simulink model "hybrid_fuzzy"  (R2020a)
settings: Solver=VariableStepAuto  StartTime=0.0  StopTime=1  RelTol=1e-3
undefined symbols (not defined in the file): DiscIntNeverNeededParam, LowerLimit, UpperLimit
libraries: powerlib x44, powerlib_extras x7, powerlib_meascontrol x6, fuzblock x2, re_lib x2, simulink x1, sdolib x1
settings Model: SimulationMode=accelerator  Creator=vardh  LastModifiedBy=vardh

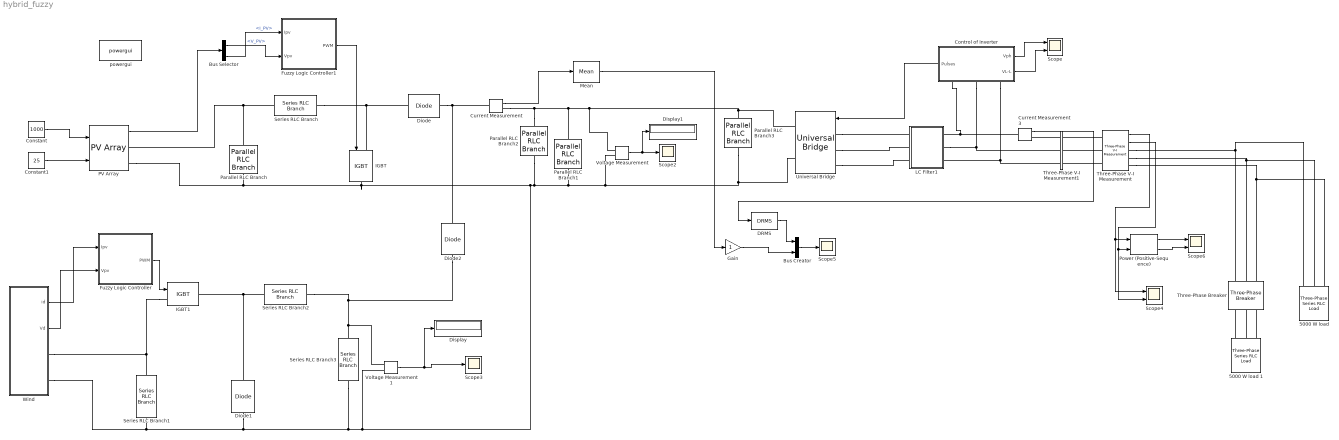
== system hybrid_fuzzy ==
  "5000 W load " : powerlib/Elements/Three-Phase Series RLC Load  LConnTagsString=A|B|C  Configuration=Y (grounded)  NominalVoltage=440  Vabc=[1e3 1e3 1e3]  Vabcp=[1e3 1e3 1e3]  NominalFrequency=50  UnbalancedPower=off  ActivePower=300e3  InductivePower=0  CapacitivePower=0  Pabc=[10e3 9e3 11e3]  QLabc=[100 90 110]  QCabc=[100 90 110]  Pabcp=[10e3 9e3 11e3]  QLabcp=[100 90 110]  QCabcp=[100 90 110]  Measurements=Branch voltages and currents  LoadType=constant PQ
  5000 W load 1 : powerlib/Elements/Three-Phase Series RLC Load  LConnTagsString=A|B|C  Configuration=Y (grounded)  NominalVoltage=440  Vabc=[1e3 1e3 1e3]  Vabcp=[1e3 1e3 1e3]  NominalFrequency=50  UnbalancedPower=off  ActivePower=300e3  InductivePower=0  CapacitivePower=0  Pabc=[10e3 9e3 11e3]  QLabc=[100 90 110]  QCabc=[100 90 110]  Pabcp=[10e3 9e3 11e3]  QLabcp=[100 90 110]  QCabcp=[100 90 110]  Measurements=Branch voltages and currents  LoadType=constant PQ
  Bus Creator : BusCreator  Inputs=2
  Bus Selector : BusSelector  OutputSignals=V_PV,I_PV
  Constant : Constant  Value=1000
  Constant1 : Constant  Value=25
  Control of Inverter : Subsystem
      settings: PortSchema="{\"entries\":[{\"content\":{\"sides\":[{\"content\":{\"connectorIds\":[\"Out2\",\"Out3\"]},\"type\":\"ConnectorPlacement.EquallySpacedRectSide\",\"uuid\":\"6e599ea3-178d-4f76-bb70-cdc4ed3450cd\"},{\"content\":{\"connectorIds\":[\"Out1\"],\"side\":\"RIGHT\"},\"type\":\"ConnectorPlacement.EquallySpacedRectSide\",\"uuid\":\"1f076554-0d11-4549-8e28-a9b47f6feaf3\"},{\"content\":{\"connectorIds\":[],\"side\":\"TOP\"},\"type\":\"ConnectorPlacement.EquallySpacedRectSide\",\"uuid\":\"86982356-7389-48f3-89f0-a125c4c11ea8\"},{\"content\":{\"connectorIds\":[\"RConn1\",\"RConn2\",\"RConn3\"],\"side\":\"BOTTOM\"},\"type\":\"ConnectorPlacement.EquallySpacedRectSide\",\"uuid\":\"f2c41feb-d46e-404e-b0df-a8035424fc9b\"}]},\"type\":\"ConnectorPlacement.EquallySpacedConnector\",\"uuid\":\"7cdef0cd-0041-4714-b9be-c27206ef597d\"}],\"packageUris\":[\"http://schema.mathworks.com/mf0/Connector/19700101\"],\"version\":\"1.0\"}"
  Current Measurement : powerlib/Measurements/Current Measurement  PhasorSimulation=off  OutputType=Complex  PSBequivalent=0
  Current Measurement3 : powerlib/Measurements/Current Measurement  PhasorSimulation=off  OutputType=Complex  PSBequivalent=0
  DRMS : sdolib/RMS Blocks/DRMS  Ts=5e-6
      settings: SourceProductBaseCode=SO
  Diode : powerlib/Power Electronics/Diode  Ron=0.001  Lon=0  Vf=0.8  IC=0  UseSnubber=0  Rs=500  Cs=250e-9  Measurements=off
  Diode1 : powerlib/Power Electronics/Diode  Ron=0.001  Lon=0  Vf=0.8  IC=0  UseSnubber=0  Rs=500  Cs=250e-9  Measurements=off
  Diode2 : powerlib/Power Electronics/Diode  Ron=0.001  Lon=0  Vf=0.8  IC=0  UseSnubber=0  Rs=500  Cs=250e-9  Measurements=off
  Display : Display
  Display1 : Display
  Fuzzy Logic Controller : Subsystem
  Fuzzy Logic Controller1 : Subsystem
  Gain : Gain
  IGBT : powerlib/Power Electronics/IGBT  Ron=0.001  Lon=0  Vf=1  Tf=1e-6  Tt=2e-6  IC=0  Rs=1e5  Cs=inf  Measurements=off
  IGBT1 : powerlib/Power Electronics/IGBT  Ron=0.001  Lon=0  Vf=1  Tf=1e-6  Tt=2e-6  IC=0  Rs=1e5  Cs=inf  Measurements=off
  LC Filter1 : Subsystem
  Mean : powerlib_meascontrol/Measurements/Mean  Freq=60  Vinit=0  Ts=5e-6
  PV Array : re_lib/Solar/PV Array  Npar=1  Nser=9  PlotType=one module @ 25 deg.C & specified irradiances  S_vec="[ 1000  800  600 ]"  Temp_C_vec="[ 45 25  ]"  ModuleName=Kyocera Solar KC200GT  PlotWhenSelected=off  Pm=200.143  Ncell=54  Voc=32.9  Isc=8.21  Vm=26.3  Im=7.61  beta_Voc_pc=-0.35502  alpha_Isc_pc=0.06  beta_Voc=-0.1168  alpha_Isc=0.004926  IL=8.2288  I0=2.3246e-10  nI=0.97736  Rsh=150.6921  Rs=0.34483  RobustModel=off  RobustCellTemperature=25  BAL=on  Tc=1e-6  Tfilter=5e-5
  Parallel RLC Branch : powerlib/Elements/Parallel RLC Branch  LConnTagsString=a  RConnTagsString=__new0  BranchType=C  Resistance=1  Inductance=1e-3  SetiL0=off  InitialCurrent=0  Capacitance=10e-6  Setx0=off  InitialVoltage=0  Measurements=None
  Parallel RLC Branch1 : powerlib/Elements/Parallel RLC Branch  LConnTagsString=a  RConnTagsString=__new0  BranchType=C  Resistance=1  Inductance=1e-3  SetiL0=off  InitialCurrent=0  Capacitance=10000e-6  Setx0=off  InitialVoltage=0  Measurements=None
  Parallel RLC Branch2 : powerlib/Elements/Parallel RLC Branch  LConnTagsString=a  RConnTagsString=__new0  BranchType=R  Resistance=30  Inductance=1e-3  SetiL0=off  InitialCurrent=0  Capacitance=1e-6  Setx0=off  InitialVoltage=0  Measurements=None
  Parallel RLC Branch3 : powerlib/Elements/Parallel RLC Branch  LConnTagsString=a  RConnTagsString=__new0  BranchType=R  Resistance=30  Inductance=1e-3  SetiL0=off  InitialCurrent=0  Capacitance=1e-6  Setx0=off  InitialVoltage=0  Measurements=None
  Power (Positive-Sequence) : powerlib_meascontrol/Measurements/Power (Positive-Sequence)  Freq=60  Vinit=[0, 0]  Iinit=[0, 0]  Ts=5e-6
      settings: SourceProductBaseCode=PS
  Scope : Scope  NumInputPorts=2
  Scope2 : Scope
  Scope3 : Scope
  Scope4 : Scope  NumInputPorts=2
  Scope5 : Scope
  Scope6 : Scope  NumInputPorts=2
  Series RLC Branch : powerlib/Elements/Series RLC Branch  LConnTagsString=__new0  RConnTagsString=__new0  BranchType=L  Resistance=1  Inductance=100e-3  SetiL0=off  InitialCurrent=0  Capacitance=1e-6  Setx0=off  InitialVoltage=0  Measurements=None
  Series RLC Branch1 : powerlib/Elements/Series RLC Branch  LConnTagsString=__new0  RConnTagsString=__new0  BranchType=C  Resistance=1  Inductance=1e-3  SetiL0=off  InitialCurrent=0  Capacitance=10e-6  Setx0=off  InitialVoltage=0  Measurements=None
  Series RLC Branch2 : powerlib/Elements/Series RLC Branch  LConnTagsString=__new0  RConnTagsString=__new0  BranchType=L  Resistance=1  Inductance=100e-3  SetiL0=off  InitialCurrent=0  Capacitance=1e-6  Setx0=off  InitialVoltage=0  Measurements=None
  Series RLC Branch3 : powerlib/Elements/Series RLC Branch  LConnTagsString=__new0  RConnTagsString=__new0  BranchType=R  Resistance=50  Inductance=1e-3  SetiL0=off  InitialCurrent=0  Capacitance=1e-6  Setx0=off  InitialVoltage=0  Measurements=None
  Three-Phase V-I Measurement : powerlib/Measurements/Three-Phase V-I Measurement  VoltageMeasurement=phase-to-phase  SetLabelV=off  LabelV=Vabc  Vpu=off  VpuLL=off  CurrentMeasurement=yes  SetLabelI=off  LabelI=Iabc  Ipu=off  Pbase=100e6  Vbase=500e3  OutputType=Complex  PhasorSimulation=off  PSBequivalent=0
  Three-Phase V-I Measurement1 : powerlib/Measurements/Three-Phase V-I Measurement  VoltageMeasurement=no  SetLabelV=off  LabelV=Vabc  Vpu=off  VpuLL=off  CurrentMeasurement=no  SetLabelI=off  LabelI=Iabc  Ipu=off  Pbase=100e6  Vbase=500e3  OutputType=Complex  PhasorSimulation=off  PSBequivalent=0
  Three-Phase Breaker : powerlib/Elements/Three-Phase Breaker  InitialState=open  SwitchA=on  SwitchB=on  SwitchC=on  SwitchTimes="[1/60  5/60]"  External=off  BreakerResistance=0.01  SnubberResistance=1e6  SnubberCapacitance=inf  Measurements=None
  Universal Bridge : powerlib/Power Electronics/Universal Bridge  Arms=3  SnubberResistance=1e5  SnubberCapacitance=inf  Device=IGBT / Diodes  Ron=1e-3  Lon=0  ForwardVoltages="[  0  0  ]"  ForwardVoltage=0  GTOparameters=[ 10e-6 , 20e-6 ]  IGBTparameters=[ 1e-6 , 2e-6 ]  Measurements=None  Measurements_2=None  converterType=Rectifier
  Voltage Measurement : powerlib/Measurements/Voltage Measurement  PhasorSimulation=off  OutputType=Complex  PSBequivalent=0
  Voltage Measurement1 : powerlib/Measurements/Voltage Measurement  PhasorSimulation=off  OutputType=Complex  PSBequivalent=0
  Wind : Subsystem
  powergui : powerlib/powergui  Priority=1  SimulationMode=Discrete  SampleTime=5e-6  frequency=60  Iterations=50  frequencyindice=0  Pbase=100e6  ErrMax=1e-4  UnitsV=kV  UnitsW=MW  buscounter=0  FunctionMessages=off  echomessages=off  EnableUseOfTLC=off  CurrentSourceSwitches=off  DisableSnubberDevices=off  DisableRonSwitches=off  DisableVfSwitches=off  DisplayEquations=off  AutomaticDiscreteSolvers=off  SolverType=Tustin/Backward Euler (TBE)  Interpol=off  ExternalGateDelay=off  methode=off  Ts=100  x0status=blocks  SPID=on  SwTol=0  HookPort=off  NonlinearTolerance=1e-4  nMaxIteration=100  ContinueOnMaxIteration=off  RestoreLinks=warning  ResistiveCurrentMeasurement=off  Frange=[0:2:500]  Ylog=off  Xlog=on  ShowGrid=off  save=off  variable=ZData  structure=0  ZoomFFT=off  StartTime=0.0  cycles=1  DisplayStyle=1  fundamental=60  FreqAxis=off  MaxFrequency=1000  frequencyindicesteady=1  RmsSteady=1  display=off
  wires:
  Bus Selector/2 -> Fuzzy Logic Controller1/1(Ipv)  "<I_PV>"
  Wind/2(Vd) -> Fuzzy Logic Controller/2(Vpv)
  Fuzzy Logic Controller1/1(PWM) -> IGBT/1
  Wind/1(id) -> Fuzzy Logic Controller/1(Ipv)
  Power (Positive-Sequence)/1 -> Scope6/1
  Bus Selector/1 -> Fuzzy Logic Controller1/2(Vpv)  "<V_PV>"
  Voltage Measurement/1 -> Display1/1, Scope2/1
  Current Measurement/1 -> Mean/1
  Control of Inverter/3(VL-L) -> Scope/2
  Fuzzy Logic Controller/1(PWM) -> IGBT1/1
  PV Array/1 -> Bus Selector/1
  Mean/1 -> Gain/1
  Current Measurement3/1 -> DRMS/1
  Three-Phase V-I Measurement/1 -> Scope4/1, Power (Positive-Sequence)/1
  Control of Inverter/1(Pulses) -> Universal Bridge/1
  Control of Inverter/2(Vph) -> Scope/1
  Power (Positive-Sequence)/2 -> Scope6/2
  Constant1/1 -> PV Array/2
  Constant/1 -> PV Array/1
  Bus Creator/1 -> Scope5/1
  Gain/1 -> Bus Creator/2
  Voltage Measurement1/1 -> Display/1, Scope3/1
  Three-Phase V-I Measurement/2 -> Scope4/2, Power (Positive-Sequence)/2
  DRMS/1 -> Bus Creator/1
  connections:
  LC Filter1/RConn3 -- Control of Inverter/RConn1 -- Three-Phase V-I Measurement1/RConn3
  Diode1/LConn1 -- Parallel RLC Branch/RConn1 -- PV Array/RConn2 -- IGBT/RConn1 -- Parallel RLC Branch1/RConn1 -- Parallel RLC Branch3/RConn1 -- Universal Bridge/RConn2 -- Voltage Measurement/LConn2 -- Parallel RLC Branch2/RConn1 -- Voltage Measurement1/LConn2 -- Series RLC Branch3/RConn1 -- Wind/RConn2 -- Series RLC Branch1/RConn1
  IGBT1/LConn1 -- Series RLC Branch1/LConn1 -- Wind/RConn1
  Voltage Measurement1/LConn1 -- Series RLC Branch2/RConn1 -- Diode2/LConn1 -- Series RLC Branch3/LConn1
  Series RLC Branch/LConn1 -- PV Array/RConn1 -- Parallel RLC Branch/LConn1
  Three-Phase V-I Measurement/RConn1 -- Three-Phase Breaker/RConn1 -- "5000 W load "/LConn1
  IGBT1/RConn1 -- Diode1/RConn1 -- Series RLC Branch2/LConn1
  Three-Phase Breaker/RConn2 -- "5000 W load "/LConn2 -- Three-Phase V-I Measurement/RConn2
  LC Filter1/RConn2 -- Control of Inverter/RConn2 -- Three-Phase V-I Measurement1/RConn2
  Current Measurement/LConn1 -- Diode/RConn1 -- Diode2/RConn1
  Parallel RLC Branch2/LConn1 -- Current Measurement/RConn1 -- Parallel RLC Branch3/LConn1 -- Universal Bridge/RConn1 -- Voltage Measurement/LConn1 -- Parallel RLC Branch1/LConn1
  LC Filter1/RConn1 -- Current Measurement3/LConn1 -- Control of Inverter/RConn3
  Three-Phase Breaker/RConn3 -- "5000 W load "/LConn3 -- Three-Phase V-I Measurement/RConn3
  Series RLC Branch/RConn1 -- Diode/LConn1 -- IGBT/LConn1
  Three-Phase V-I Measurement/LConn2 -- Three-Phase V-I Measurement1/LConn2
  Universal Bridge/LConn1 -- LC Filter1/LConn1
  Three-Phase V-I Measurement/LConn1 -- Three-Phase V-I Measurement1/LConn1
  Three-Phase V-I Measurement/LConn3 -- Three-Phase V-I Measurement1/LConn3
  5000 W load 1/LConn1 -- Three-Phase Breaker/LConn1
  Universal Bridge/LConn3 -- LC Filter1/LConn3
  Three-Phase V-I Measurement1/RConn1 -- Current Measurement3/RConn1
  5000 W load 1/LConn3 -- Three-Phase Breaker/LConn3
  Universal Bridge/LConn2 -- LC Filter1/LConn2
  5000 W load 1/LConn2 -- Three-Phase Breaker/LConn2

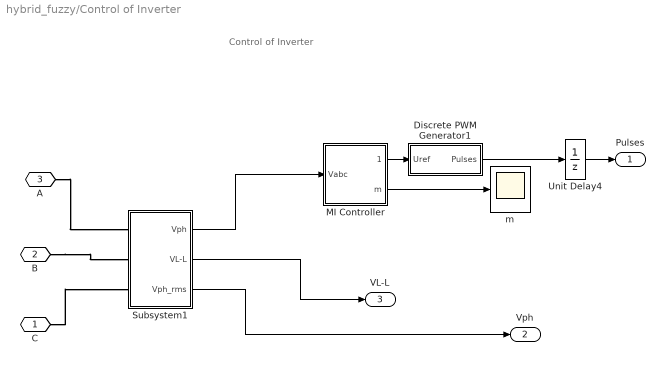
== system hybrid_fuzzy/Control of Inverter ==
  note: Control of Inverter
  Discrete PWM Generator1 : Subsystem  AncestorBlock=|  DialogController=POWERSYS.PowerSysDialog  mask(Discrete PWM Generator){GeneratorMode=3-arm  bridge (6 pulses), Fc=10000, Ts=5e-6, Internal=off, mIndex=0.99, Freq=50, Phase=0}
      | powerlib_extras/Discrete 
      | Control Blocks/Discrete
      | PWM Generator
      mask prompts: GeneratorMode "Generator Mode"; Fc "Carrier frequency (Hz):"; Ts "Sample time:"; Internal "Internal generation of modulating signal(s)"; mIndex "Modulation index  (0<m<1) :"; Freq "Frequency of output voltage (Hz)"; Phase "Phase of output voltage (degrees)"
      mask help:
      | This discrete block generates pulses for carrier-based PWM (Pulse Width Modulation), self-commutated IGBTs,GTOs or FETs bridges.
      |
      | Depending on the number of bridge arms selected in the "Generator Mode" parameter, the block can be used either for single-phase or three-phase PWM control.
      mask init:
      | powericon('psbcallbacks',gcb,'Discrete PWM Generator');
      | if Freq==0
      |     Phase=90;
      | end
      | switch GeneratorMode
      | case 1,
      |     Internal_Phase=0;
      |    Signal_PortWidth=1;
      |    Select1_Elements=[1 2];
      |    Select1_PortWidth=2;
      |    Select3_Elements=[1 2];
      |    Select3_PortWidth=4;
      | case 2,
      |     Internal_Phase=0;
      |     Signal_PortWidth=1;
      |     Select1_Elements=[1 2];
      |     Select1_PortWidth=2;
      |     Select3_Elements=[1 2 3 4];
      |     Select3_PortWidth=4;
      | case 3,
      |     Internal_Phase=[0 -2*pi/3 2*pi/3];
      |     Signal_PortWidth=3;
      |     Select1_Elements=[1 4 2 5 3 6];
      |     Select1_PortWidth=6;
      |    Select3_Elements=[1 2 3 4 5 6];
      |    Select3_PortWidth=12;
      | case 4,
      |     Internal_Phase=[0 -2*pi/3 2*pi/3];
      |     Signal_PortWidth=3;
      |     Select1_Elements=[1 4 2 5 3 6];
      |     Select1_PortWidth=6;
      |    Select3_Elements=[1 2 3 4 5 6 7 8 9 10 11 12];
      |    Select3_PortWidth=12;
      | end
      | power_initmask();
      mask Help:
      | The output pulses are a vector (with values=0 or 1). Depending on the selected "Generator Mode", the output vector contains:
      | For a 1-arm  bridge: Two pulses. Pulse 1 is for the upper switch and pulse 2 is for the lower switch.
      | For a 2-arm  bridge: Four pulses. Pulses 1 and 3 are respectively for the upper switches of the first and second arm. Pulses 2 and 4 are for the lower switches.
      | For a 3-arm  bridge: Six pulses. Pulses 1,3 and 5 are respectively for the upper switches of the first,second and third arm. Pulses 2,4 and 6 are for the lower switches.
      | For double 3-arm bridges: Twelve pulses.The first six pulses (pulses 1 to 6) must be sent to the first 3-arm bridge and the last six (pulses 7 to 12) to the second 3-arm bridge.
      | 
      | By selecting "Internal generation" you can can control the modulation index m, frequency and phase of the output voltage  from the internal parameters (m, Freq and Phase). Otherwise, external signals are used for pulse generation. The width of the input vector must be 1 for single phase bridges ( 1-arm or 2-arm)  and 3 for 3-phase bridges  (single or double bridge).
      mask TypeOptions GeneratorMode: 1-arm  bridge (2 pulses) | 2-arm  bridge (4 pulses) | 3-arm  bridge (6 pulses) | Double 3-arm  bridges (12 pulses)
      mask Callback Internal: powericon('psbcallbacks',gcb,'Discrete PWM Generator',[]);
  MI Controller : Subsystem
  Subsystem1 : Subsystem
  Unit Delay4 : UnitDelay  SampleTime=5e-6  HasFrameUpgradeWarning=on
  m : Scope
  C : PMIOPort  Side=Right
  B : PMIOPort  Port=2  Side=Right
  A : PMIOPort  Port=3  Side=Right
  Pulses : Outport  VectorParamsAs1DForOutWhenUnconnected=off
  Vph : Outport  Port=2  VectorParamsAs1DForOutWhenUnconnected=off
  VL-L : Outport  Port=3  VectorParamsAs1DForOutWhenUnconnected=off
  wires:
  MI Controller/2(m) -> m/1
  Unit Delay4/1 -> Pulses/1
  Subsystem1/1(Vph) -> MI Controller/1(Vabc)
  Subsystem1/2(VL-L) -> VL-L/1
  Subsystem1/3(Vph_rms) -> Vph/1
  Discrete PWM Generator1/1(Pulses) -> Unit Delay4/1
  MI Controller/1(Vabc_inv) -> Discrete PWM Generator1/1(Uref)
  connections:
  A/RConn1 -- Subsystem1/LConn1
  B/RConn1 -- Subsystem1/LConn2
  C/RConn1 -- Subsystem1/LConn3

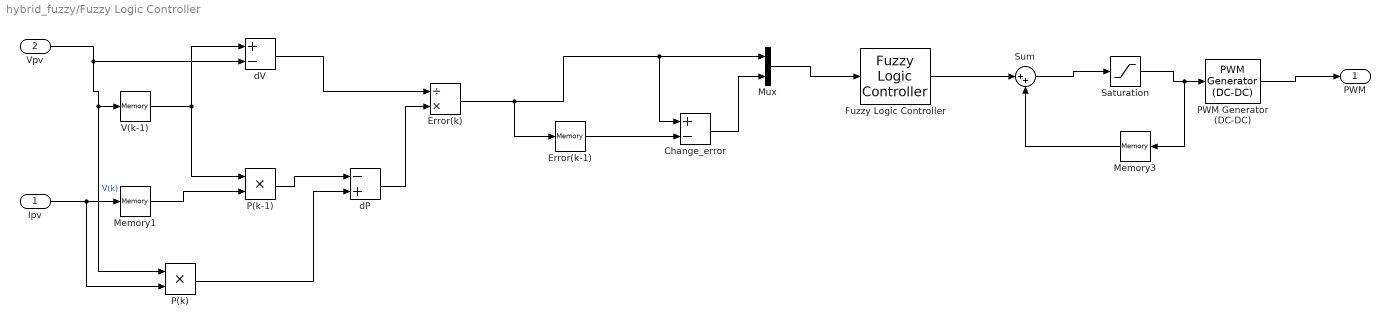
== system hybrid_fuzzy/Fuzzy Logic Controller ==
  Ipv : Inport
  Vpv : Inport  Port=2
  Change_error : Sum  Inputs=+-
  Error(k) : Product  Inputs=/*
  Error(k-1) : Memory
  Fuzzy Logic Controller : fuzblock/Fuzzy Logic  Controller  FIS='fuzzy_ctrl_other.fis'  OutputSampleNumber=101  DataType=double  FuzzifiedInputs=off  RuleFiringStrengths=off  RuleOutputs=off  AggregatedOutputs=off  SimulateUsing=Interpreted execution  OutOfRangeInputValueMessage=none  NoRuleFiredMessage=none  EmptyOutputFuzzySetMessage=none
  Memory1 : Memory
  Memory3 : Memory
  Mux : Mux  Inputs=2
  P(k) : Product
  P(k-1) : Product
  PWM Generator (DC-DC) : powerlib_meascontrol/Pulse & Signal Generators/PWM Generator (DC-DC)  Fsw=20000  Ts=0
  Saturation : Saturate
  Sum : Sum  Inputs=|++
  V(k-1) : Memory
  dP : Sum  Inputs=-+
  dV : Sum  Inputs=+-
  PWM : Outport
  wires:
  Vpv/1 -> P(k)/1, V(k-1)/1, dV/2  "V(k)"
  V(k-1)/1 -> dV/1, P(k-1)/1
  Ipv/1 -> P(k)/2, Memory1/1
  Memory1/1 -> P(k-1)/2
  P(k)/1 -> dP/2
  P(k-1)/1 -> dP/1
  dV/1 -> Error(k)/1
  dP/1 -> Error(k)/2
  Error(k)/1 -> Error(k-1)/1, Change_error/1, Mux/1
  Error(k-1)/1 -> Change_error/2
  Mux/1 -> Fuzzy Logic Controller/1
  Change_error/1 -> Mux/2
  Fuzzy Logic Controller/1 -> Sum/1
  Memory3/1 -> Sum/2
  Sum/1 -> Saturation/1
  Saturation/1 -> Memory3/1, PWM Generator (DC-DC)/1
  PWM Generator (DC-DC)/1 -> PWM/1

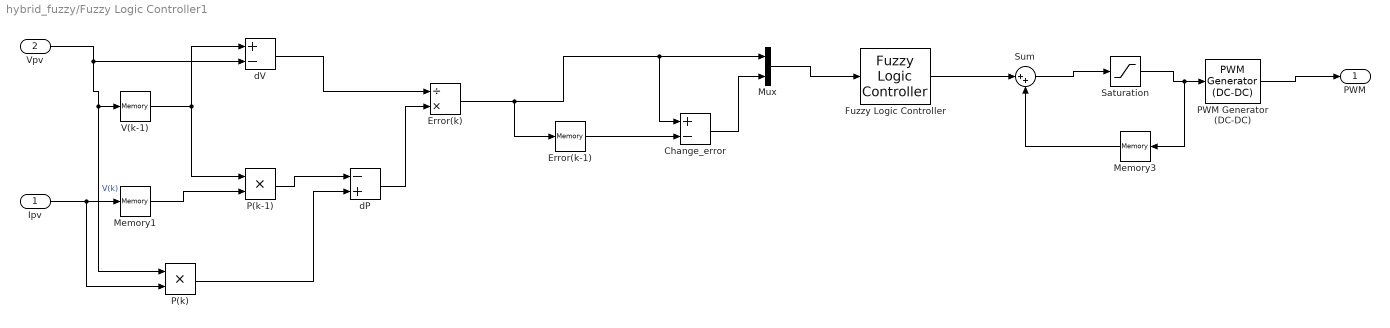
== system hybrid_fuzzy/Fuzzy Logic Controller1 ==
  Ipv : Inport
  Vpv : Inport  Port=2
  Change_error : Sum  Inputs=+-
  Error(k) : Product  Inputs=/*
  Error(k-1) : Memory
  Fuzzy Logic Controller : fuzblock/Fuzzy Logic  Controller  FIS='fuzzy_ctrl_other.fis'  OutputSampleNumber=101  DataType=double  FuzzifiedInputs=off  RuleFiringStrengths=off  RuleOutputs=off  AggregatedOutputs=off  SimulateUsing=Interpreted execution  OutOfRangeInputValueMessage=none  NoRuleFiredMessage=none  EmptyOutputFuzzySetMessage=none
  Memory1 : Memory
  Memory3 : Memory
  Mux : Mux  Inputs=2
  P(k) : Product
  P(k-1) : Product
  PWM Generator (DC-DC) : powerlib_meascontrol/Pulse & Signal Generators/PWM Generator (DC-DC)  Fsw=20000  Ts=0
  Saturation : Saturate
  Sum : Sum  Inputs=|++
  V(k-1) : Memory
  dP : Sum  Inputs=-+
  dV : Sum  Inputs=+-
  PWM : Outport
  wires:
  PWM Generator (DC-DC)/1 -> PWM/1
  Saturation/1 -> PWM Generator (DC-DC)/1, Memory3/1
  Sum/1 -> Saturation/1
  Memory3/1 -> Sum/2
  Fuzzy Logic Controller/1 -> Sum/1
  Change_error/1 -> Mux/2
  Mux/1 -> Fuzzy Logic Controller/1
  Error(k-1)/1 -> Change_error/2
  Error(k)/1 -> Mux/1, Change_error/1, Error(k-1)/1
  dP/1 -> Error(k)/2
  dV/1 -> Error(k)/1
  P(k-1)/1 -> dP/1
  P(k)/1 -> dP/2
  Memory1/1 -> P(k-1)/2
  Ipv/1 -> Memory1/1, P(k)/2
  V(k-1)/1 -> P(k-1)/1, dV/1
  Vpv/1 -> dV/2, V(k-1)/1, P(k)/1  "V(k)"

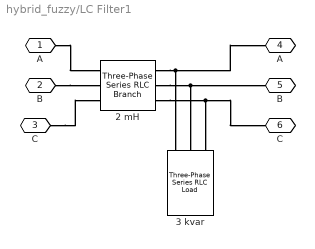
== system hybrid_fuzzy/LC Filter1 ==
  "2 mH " : powerlib/Elements/Three-Phase Series RLC Branch  LConnTagsString=A|B|C  RConnTagsString=A|B|C  BranchType=L  Resistance=0  Inductance=2e-3  Capacitance=inf  Measurements=None
  3 kvar : powerlib/Elements/Three-Phase Series RLC Load  LConnTagsString=A|B|C  Configuration=Y (grounded)  NominalVoltage=440  Vabc=[1e3 1e3 1e3]  Vabcp=[1e3 1e3 1e3]  NominalFrequency=50  UnbalancedPower=off  ActivePower=0  InductivePower=0  CapacitivePower=3e3  Pabc=[10e3 9e3 11e3]  QLabc=[100 90 110]  QCabc=[100 90 110]  Pabcp=[10e3 9e3 11e3]  QLabcp=[100 90 110]  QCabcp=[100 90 110]  Measurements=None  LoadType=constant Z
  A : PMIOPort  Side=Left
  B : PMIOPort  Port=2  Side=Left
  C : PMIOPort  Port=3  Side=Left
  "A " : PMIOPort  Port=4  Side=Right
  "B " : PMIOPort  Port=5  Side=Right
  "C " : PMIOPort  Port=6  Side=Right
  connections:
  B/RConn1 -- "2 mH "/LConn2
  A/RConn1 -- "2 mH "/LConn1
  C/RConn1 -- "2 mH "/LConn3
  "2 mH "/RConn1 -- "A "/RConn1 -- 3 kvar/LConn1
  "2 mH "/RConn2 -- "B "/RConn1 -- 3 kvar/LConn2
  "2 mH "/RConn3 -- "C "/RConn1 -- 3 kvar/LConn3

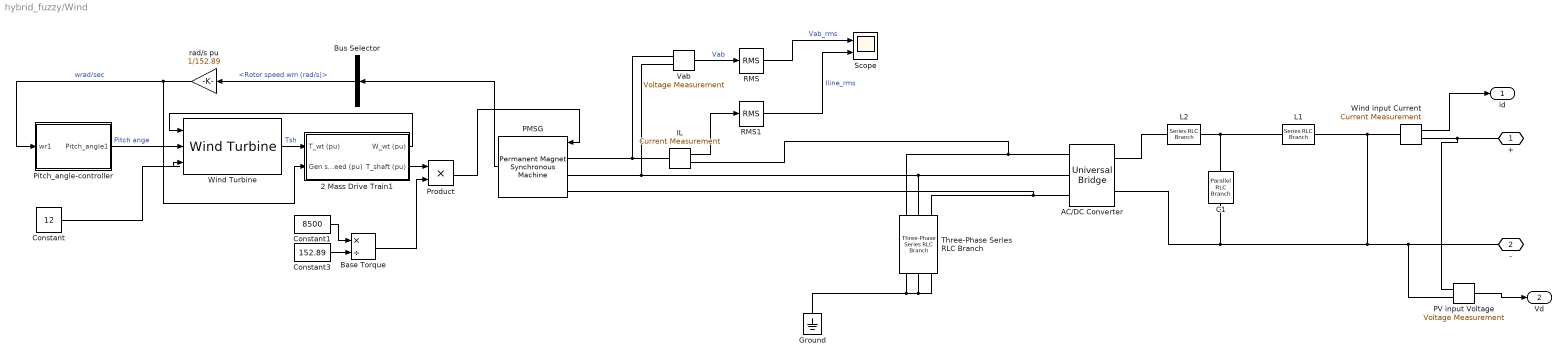
== system hybrid_fuzzy/Wind ==
  2 Mass Drive Train1 : Subsystem
  AC/DC Converter : powerlib/Power Electronics/Universal Bridge  Arms=3  SnubberResistance=1e5  SnubberCapacitance=inf  Device=Diodes  Ron=1e-3  Lon=0  ForwardVoltages="[  0  0  ]"  ForwardVoltage=0  GTOparameters=[ 10e-6 , 20e-6 ]  IGBTparameters=[ 1e-6 , 2e-6 ]  Measurements=None  Measurements_2=None  converterType=Rectifier
  Base Torque : Product  Inputs=*/  RndMeth=Zero
  Bus Selector : BusSelector  OutputSignals=Rotor speed wm (rad/s)
  C1 : powerlib/Elements/Parallel RLC Branch  LConnTagsString=a  RConnTagsString=__new0  BranchType=C  Resistance=1.0  Inductance=1.0  SetiL0=off  InitialCurrent=0  Capacitance=1000e-06  Setx0=off  InitialVoltage=650  Measurements=None
  Constant : Constant  Value=12
  Constant1 : Constant  Value=8500
  Constant3 : Constant  Value=152.89
  Ground : powerlib/Elements/Ground  LConnTagsString=a
  IL : powerlib/Measurements/Current Measurement  PhasorSimulation=off  OutputType=Complex  PSBequivalent=0
  L1 : powerlib/Elements/Series RLC Branch  LConnTagsString=__new0  RConnTagsString=__new0  BranchType=L  Resistance=1.0  Inductance=2e-3  SetiL0=off  InitialCurrent=0  Capacitance=1.0  Setx0=off  InitialVoltage=0  Measurements=None
  L2 : powerlib/Elements/Series RLC Branch  LConnTagsString=__new0  RConnTagsString=__new0  BranchType=L  Resistance=1.0  Inductance=2e-3  SetiL0=off  InitialCurrent=0  Capacitance=1.0  Setx0=off  InitialVoltage=0  Measurements=None
  PMSG : powerlib/Machines/Permanent Magnet Synchronous Machine  NbPhases=3  FluxDistribution=Sinusoidal  RotorType=Salient-pole  MechanicalLoad=Torque Tm  PresetModel=No  ShowDetailedParameters=on  MeasurementBus=off  Resistance=0.425  Inductance=8.5e-3  dqInductances=[0.0082 0.0082]  La=0.000835  MachineConstant=Flux linkage established by magnets (V.s)  Flux=0.433  VoltageCst=392.6876  TorqueCst=3.2475  Flat=120  Mechanical=[0.01197 0.001189 5]  PolePairs=5  InitialConditions=[0,0, 0,0]  InitialConditions5ph=[0 0 0 0 0 0]  RefAngle=90 degrees behind phase A axis (modified Park)  IterativeDiscreteModel=Trapezoidal non iterative  TsBlock=-1  TsPowergui=0
  PV input Voltage : powerlib/Measurements/Voltage Measurement  PhasorSimulation=off  OutputType=Complex  PSBequivalent=0
  Pitch_angle-controller : Subsystem
  Product : Product  RndMeth=Zero
  RMS : powerlib_meascontrol/Measurements/RMS  TrueRMS=off  Freq=50  RMSInit=0  Ts=20e-6
  RMS1 : powerlib_meascontrol/Measurements/RMS  TrueRMS=off  Freq=50  RMSInit=0  Ts=20e-6
  Scope : Scope  NumInputPorts=2
  Three-Phase Series RLC Branch : powerlib/Elements/Three-Phase Series RLC Branch  LConnTagsString=A|B|C  RConnTagsString=A|B|C  BranchType=R  Resistance=800  Inductance=1e-3  Capacitance=1e-6  Measurements=None
  Vab : powerlib/Measurements/Voltage Measurement  PhasorSimulation=off  OutputType=Complex  PSBequivalent=0
  Wind Turbine : re_lib/Wind Generation/Wind Turbine  Pnom=8.5e3  Pelec_base=8.5e3/0.9  wind_base=12  P_wind_base=0.8  speed_nom=1  pitch_angle=0  c1_c6="[0.51763          116          0.4            5           21     0.006795]"  cp_nom=0.48  lambda_nom=8.1
      settings: SourceProductBaseCode=PS
  Wind input Current : powerlib/Measurements/Current Measurement  PhasorSimulation=off  OutputType=Complex  PSBequivalent=0
  rad/s pu : Gain  Gain=1/152.89  SaturateOnIntegerOverflow=on  OutDataTypeStr=Inherit: Same as input  ParamDataTypeStr=Inherit: Same as input
  + : PMIOPort  Side=Right
  - : PMIOPort  Port=2  Side=Right
  id : Outport
  Vd : Outport  Port=2
  wires:
  IL/1 -> RMS1/1
  Constant/1 -> Wind Turbine/3
  Product/1 -> PMSG/1
  rad/s pu/1 -> Pitch_angle-controller/1(wr1), 2 Mass Drive Train1/2(Gen speed (pu))  "wrad/sec"
  2 Mass Drive Train1/1(W_wt (pu)) -> Wind Turbine/1
  Bus Selector/1 -> rad/s pu/1  "<Rotor speed wm (rad/s)>"
  Vab/1 -> RMS/1  "Vab"
  2 Mass Drive Train1/2(T_shaft (pu)) -> Product/1
  Constant3/1 -> Base Torque/2
  RMS/1 -> Scope/1  "Vab_rms"
  Pitch_angle-controller/1(Pitch_angle1) -> Wind Turbine/2  "Pitch ange"
  RMS1/1 -> Scope/2  "Iline_rms"
  PMSG/1 -> Bus Selector/1
  Wind Turbine/1 -> 2 Mass Drive Train1/1(T_wt (pu))  "Tsh"
  Constant1/1 -> Base Torque/1
  Base Torque/1 -> Product/2
  PV input Voltage/1 -> Vd/1
  Wind input Current/1 -> id/1
  connections:
  Three-Phase Series RLC Branch/LConn2 -- PMSG/LConn2 -- Vab/LConn2 -- AC/DC Converter/LConn2
  Three-Phase Series RLC Branch/LConn3 -- PMSG/LConn3 -- AC/DC Converter/LConn3
  Vab/LConn1 -- PMSG/LConn1 -- IL/LConn1
  Three-Phase Series RLC Branch/LConn1 -- IL/RConn1 -- AC/DC Converter/LConn1
  PV input Voltage/LConn1 -- +/RConn1 -- Wind input Current/RConn1
  C1/RConn1 -- AC/DC Converter/RConn2 -- -/RConn1 -- PV input Voltage/LConn2 -- Wind input Current/LConn1 -- L1/RConn1
  L1/LConn1 -- C1/LConn1 -- L2/RConn1
  Three-Phase Series RLC Branch/RConn1 -- Three-Phase Series RLC Branch/RConn3 -- Three-Phase Series RLC Branch/RConn2 -- Ground/LConn1
  L2/LConn1 -- AC/DC Converter/RConn1

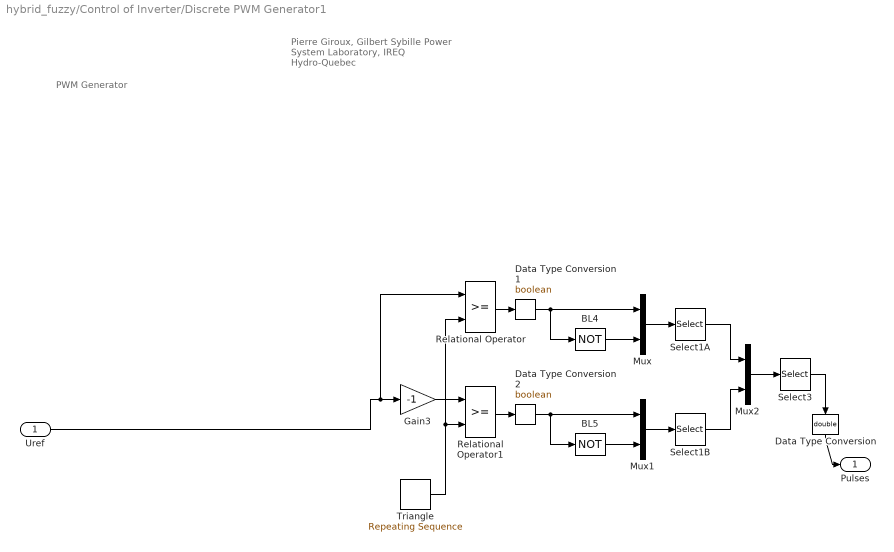
== system hybrid_fuzzy/Control of Inverter/Discrete PWM Generator1 ==
  note: Pierre Giroux, Gilbert Sybille
      | Power System Laboratory, IREQ
      | Hydro-Quebec
  note: PWM Generator
  Uref : Inport
  BL4 : Logic  Operator=NOT  Inputs=1
  BL5 : Logic  Operator=NOT  Inputs=1
  Data Type Conversion : DataTypeConversion  OutDataTypeStr=double  SaturateOnIntegerOverflow=on  RndMeth=Zero
  Data Type Conversion1 : DataTypeConversion  OutDataTypeStr=boolean  SaturateOnIntegerOverflow=on  RndMeth=Zero
  Data Type Conversion2 : DataTypeConversion  OutDataTypeStr=boolean  SaturateOnIntegerOverflow=on  RndMeth=Zero
  Gain3 : Gain  Gain=-1  SaturateOnIntegerOverflow=on  OutDataTypeStr=Inherit: Same as input  ParamDataTypeStr=Inherit: Same as input
  Mux : Mux  Inputs=2
  Mux1 : Mux  Inputs=2
  Mux2 : Mux  Inputs=2
  Relational Operator : RelationalOperator  RndMeth=Nearest  InputSameDT=on
  Relational Operator1 : RelationalOperator  RndMeth=Nearest  InputSameDT=on
  Select1A : Selector  InputPortWidth=Select1_PortWidth  IndexOptions=Index vector (dialog)  Indices=Select1_Elements  OutputSizes=1
  Select1B : Selector  InputPortWidth=Select1_PortWidth  IndexOptions=Index vector (dialog)  Indices=Select1_Elements  OutputSizes=1
  Select3 : Selector  InputPortWidth=Select3_PortWidth  IndexOptions=Index vector (dialog)  Indices=Select3_Elements  OutputSizes=1
  Triangle : simulink/Sources/Repeating Sequence  rep_seq_t=[0 1/Fc/4 3/Fc/4 1/Fc]  rep_seq_y=[0 -1 1 0]
  Pulses : Outport  VectorParamsAs1DForOutWhenUnconnected=off
  wires:
  Mux2/1 -> Select3/1
  Select1B/1 -> Mux2/2
  Select1A/1 -> Mux2/1
  Mux1/1 -> Select1B/1
  Mux/1 -> Select1A/1
  BL5/1 -> Mux1/2
  BL4/1 -> Mux/2
  Gain3/1 -> Relational Operator1/1
  Triangle/1 -> Relational Operator1/2, Relational Operator/2
  Uref/1 -> Relational Operator/1, Gain3/1
  Select3/1 -> Data Type Conversion/1
  Data Type Conversion/1 -> Pulses/1
  Relational Operator/1 -> Data Type Conversion1/1
  Data Type Conversion1/1 -> BL4/1, Mux/1
  Relational Operator1/1 -> Data Type Conversion2/1
  Data Type Conversion2/1 -> BL5/1, Mux1/1

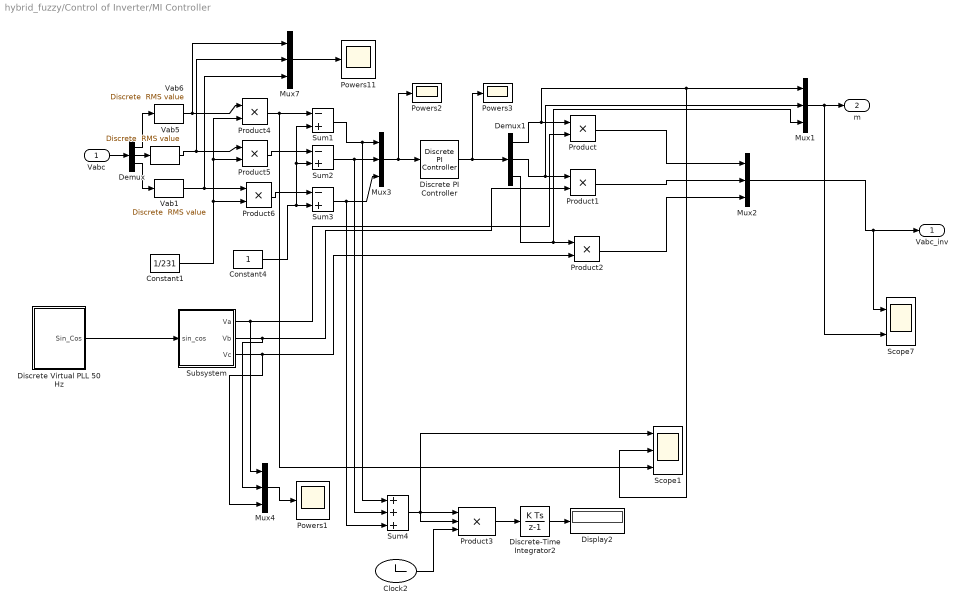
== system hybrid_fuzzy/Control of Inverter/MI Controller ==
  Vabc : Inport
  Clock2 : Clock
  Constant1 : Constant  Value=1/231
  Constant4 : Constant
  Demux : Demux  Outputs=3
  Demux1 : Demux  Outputs=3
  Discrete PI Controller : powerlib_extras/Discrete  Control Blocks/Discrete PI Controller  Kp=2  Ki=42  Par_Limits=[1.5 -1]  Init=0  Ts=5e-6
  Discrete Virtual PLL 50 Hz : Subsystem  AncestorBlock=|  DialogController=POWERSYS.PowerSysDialog  mask(Discrete Virtual PLL){Freq=50, Phase=0, Ts=5e-6}
      | powerlib_extras/Discrete 
      | Control Blocks/Discrete
      | Virtual PLL
      mask prompts: Freq "Frequency (Hz):"; Phase "Phase (degrees):"; Ts "Sample time:"
      mask help:
      | This virtual PLL has no input signal. The block simulates the outputs of an actual PLL by  using the parameters specified in the mask.
      |
      | Output 1: Frequency (Hz)
      | Output 2: Vectorized output  [sin(wt)  cos(wt)]
      | Output 3: wt in rad/s (varying from 0 to 2*pi)
      mask init:
      | power_initmask();
      mask Help: This block is part of a subset of blocks in the Extras library that does not have documentation associated with it, other than the block mask description.
      mask Display: disp('')
  Discrete-Time Integrator2 : DiscreteIntegrator  SampleTime=5e-6  UpperSaturationLimit=UpperLimit  LowerSaturationLimit=LowerLimit  ICPrevOutput=DiscIntNeverNeededParam  ICPrevScaledInput=DiscIntNeverNeededParam
  Display2 : Display
  Mux{1..4,7} (5 alike) : Mux  Inputs=3
  Powers{1..3,11} (4 alike) : Scope
  Product{,1..2,4..6} (6 alike) : Product  RndMeth=Zero
  Product3 : Product  Inputs=3  InputSameDT=on  RndMeth=Zero  SaturateOnIntegerOverflow=on  OutDataTypeStr=Inherit: Same as first input
  Scope1 : Scope  NumInputPorts=3
  Scope7 : Scope  NumInputPorts=2
  Subsystem : Subsystem
  Sum1 : Sum  Inputs=-+  InputSameDT=on  SaturateOnIntegerOverflow=on  OutDataTypeStr=Inherit: Same as first input
  Sum2 : Sum  Inputs=-+  InputSameDT=on  SaturateOnIntegerOverflow=on  OutDataTypeStr=Inherit: Same as first input
  Sum3 : Sum  Inputs=-+  InputSameDT=on  SaturateOnIntegerOverflow=on  OutDataTypeStr=Inherit: Same as first input
  Sum4 : Sum  Inputs=+++  InputSameDT=on  SaturateOnIntegerOverflow=on  OutDataTypeStr=Inherit: Same as first input
  Vab1 : powerlib_extras/Discrete Measurements/Discrete  RMS value  Freq=50  Mag_Init=0  Ts=5e-6
      settings: SourceProductBaseCode=PS
  Vab5 : powerlib_extras/Discrete Measurements/Discrete  RMS value  Freq=50  Mag_Init=0  Ts=5e-6
      settings: SourceProductBaseCode=PS
  Vab6 : powerlib_extras/Discrete Measurements/Discrete  RMS value  Freq=50  Mag_Init=0  Ts=5e-6
      settings: SourceProductBaseCode=PS
  Vabc_inv : Outport  VectorParamsAs1DForOutWhenUnconnected=off
  m : Outport  Port=2  VectorParamsAs1DForOutWhenUnconnected=off
  wires:
  Mux2/1 -> Vabc_inv/1, Scope7/1
  Product/1 -> Mux2/1
  Product1/1 -> Mux2/2
  Product2/1 -> Mux2/3
  Mux1/1 -> m/1, Scope7/2
  Vab5/1 -> Mux7/2, Product5/1
  Vab1/1 -> Mux7/3, Product6/1
  Constant4/1 -> Sum3/2, Sum2/2, Sum1/2
  Sum1/1 -> Mux3/1, Sum4/1
  Vabc/1 -> Demux/1
  Demux/1 -> Vab6/1
  Demux/2 -> Vab5/1
  Demux/3 -> Vab1/1
  Product3/1 -> Discrete-Time Integrator2/1
  Clock2/1 -> Product3/3
  Discrete-Time Integrator2/1 -> Display2/1
  Sum2/1 -> Mux3/2, Sum4/2
  Sum3/1 -> Mux3/3, Sum4/3
  Mux3/1 -> Powers2/1, Discrete PI Controller/1
  Discrete PI Controller/1 -> Powers3/1, Demux1/1
  Demux1/1 -> Product/1, Mux1/1, Scope1/2
  Demux1/2 -> Product1/1, Mux1/2
  Demux1/3 -> Product2/1, Mux1/3
  Product4/1 -> Sum1/1, Scope1/3
  Product5/1 -> Sum2/1
  Product6/1 -> Sum3/1
  Vab6/1 -> Mux7/1, Product4/1
  Mux7/1 -> Powers11/1
  Discrete Virtual PLL 50 Hz/1(Sin_Cos) -> Subsystem/1(sin_cos)
  Subsystem/1(Va) -> Product/2, Mux4/1
  Subsystem/2(Vb) -> Product1/2, Mux4/2
  Subsystem/3(Vc) -> Product2/2, Mux4/3
  Mux4/1 -> Powers1/1
  Constant1/1 -> Product6/2, Product5/2, Product4/2
  Sum4/1 -> Product3/1, Product3/2, Scope1/1

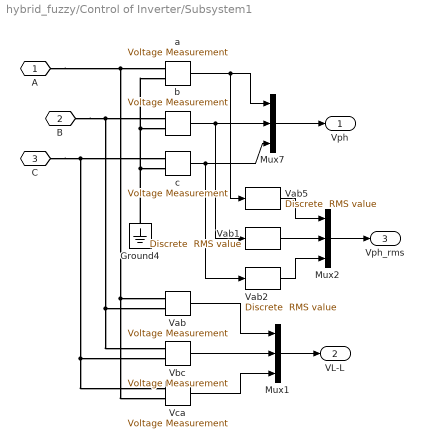
== system hybrid_fuzzy/Control of Inverter/Subsystem1 ==
  Ground4 : powerlib/Elements/Ground  LConnTagsString=a
  Mux1 : Mux  Inputs=3
  Mux2 : Mux  Inputs=3
  Mux7 : Mux  Inputs=3
  Vab : powerlib/Measurements/Voltage Measurement  Tag=PoWeRsYsTeMmEaSuReMeNt  PhasorSimulation=off  OutputType=Magnitude  PSBequivalent=0
  Vab1 : powerlib_extras/Discrete Measurements/Discrete  RMS value  Freq=50  Mag_Init=0  Ts=5e-6
      settings: SourceProductBaseCode=PS
  Vab2 : powerlib_extras/Discrete Measurements/Discrete  RMS value  Freq=50  Mag_Init=0  Ts=5e-6
      settings: SourceProductBaseCode=PS
  Vab5 : powerlib_extras/Discrete Measurements/Discrete  RMS value  Freq=50  Mag_Init=0  Ts=5e-6
      settings: SourceProductBaseCode=PS
  Vbc : powerlib/Measurements/Voltage Measurement  Tag=PoWeRsYsTeMmEaSuReMeNt  PhasorSimulation=off  OutputType=Magnitude  PSBequivalent=0
  Vca : powerlib/Measurements/Voltage Measurement  Tag=PoWeRsYsTeMmEaSuReMeNt  PhasorSimulation=off  OutputType=Magnitude  PSBequivalent=0
  a : powerlib/Measurements/Voltage Measurement  Tag=PoWeRsYsTeMmEaSuReMeNt  PhasorSimulation=off  OutputType=Magnitude  PSBequivalent=0
  b : powerlib/Measurements/Voltage Measurement  Tag=PoWeRsYsTeMmEaSuReMeNt  PhasorSimulation=off  OutputType=Magnitude  PSBequivalent=0
  c : powerlib/Measurements/Voltage Measurement  Tag=PoWeRsYsTeMmEaSuReMeNt  PhasorSimulation=off  OutputType=Magnitude  PSBequivalent=0
  A : PMIOPort  Side=Left
  B : PMIOPort  Port=2  Side=Left
  C : PMIOPort  Port=3  Side=Left
  Vph : Outport  VectorParamsAs1DForOutWhenUnconnected=off
  VL-L : Outport  Port=2  VectorParamsAs1DForOutWhenUnconnected=off
  Vph_rms : Outport  Port=3  VectorParamsAs1DForOutWhenUnconnected=off
  wires:
  a/1 -> Mux7/1, Vab5/1
  b/1 -> Mux7/2, Vab1/1
  c/1 -> Mux7/3, Vab2/1
  Mux7/1 -> Vph/1
  Vab/1 -> Mux1/1
  Vbc/1 -> Mux1/2
  Vca/1 -> Mux1/3
  Mux1/1 -> VL-L/1
  Vab5/1 -> Mux2/1
  Vab1/1 -> Mux2/2
  Vab2/1 -> Mux2/3
  Mux2/1 -> Vph_rms/1
  connections:
  Ground4/LConn1 -- c/LConn2 -- b/LConn2 -- a/LConn2
  A/RConn1 -- a/LConn1 -- Vab/LConn1 -- Vca/LConn2
  B/RConn1 -- b/LConn1 -- Vab/LConn2 -- Vbc/LConn1
  C/RConn1 -- c/LConn1 -- Vbc/LConn2 -- Vca/LConn1

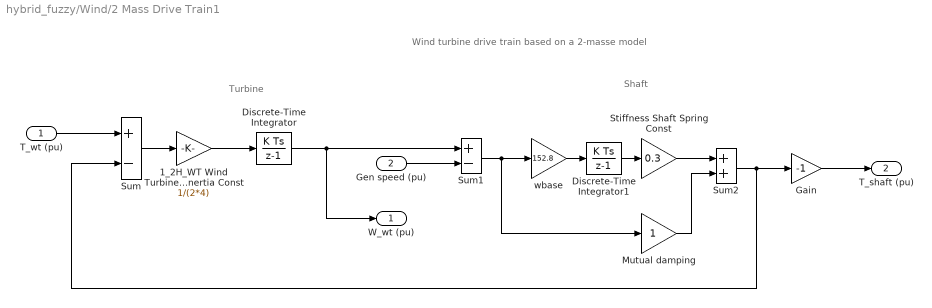
== system hybrid_fuzzy/Wind/2 Mass Drive Train1 ==
  note: Wind turbine drive train based on a 2-masse model
  note: Turbine
  note: Shaft
  T_wt (pu) : Inport
  Gen speed (pu) : Inport  Port=2
  1_2H_WT Wind Turbine Inertia Const : Gain  Gain=1/(2*4)  SaturateOnIntegerOverflow=on  OutDataTypeStr=Inherit: Same as input  ParamDataTypeStr=Inherit: Same as input
  Discrete-Time Integrator : DiscreteIntegrator  InitialCondition=1  SampleTime=20e-6  ICPrevOutput=DiscIntNeverNeededParam  ICPrevScaledInput=DiscIntNeverNeededParam
  Discrete-Time Integrator1 : DiscreteIntegrator  InitialCondition=1/0.3  SampleTime=20e-6  UpperSaturationLimit=4  LowerSaturationLimit=-4  ICPrevOutput=DiscIntNeverNeededParam  ICPrevScaledInput=DiscIntNeverNeededParam
  Gain : Gain  Gain=-1  SaturateOnIntegerOverflow=on  OutDataTypeStr=Inherit: Same as input  ParamDataTypeStr=Inherit: Same as input
  Mutual damping : Gain  SaturateOnIntegerOverflow=on  OutDataTypeStr=Inherit: Same as input  ParamDataTypeStr=Inherit: Same as input
  Stiffness Shaft Spring Const : Gain  Gain=0.3  SaturateOnIntegerOverflow=on  OutDataTypeStr=Inherit: Same as input  ParamDataTypeStr=Inherit: Same as input
  Sum : Sum  Inputs=+-  InputSameDT=on  SaturateOnIntegerOverflow=on  OutDataTypeStr=Inherit: Same as first input
  Sum1 : Sum  Inputs=+-  InputSameDT=on  SaturateOnIntegerOverflow=on  OutDataTypeStr=Inherit: Same as first input
  Sum2 : Sum  InputSameDT=on  SaturateOnIntegerOverflow=on  OutDataTypeStr=Inherit: Same as first input
  wbase : Gain  Gain=152.8  SaturateOnIntegerOverflow=on  OutDataTypeStr=Inherit: Same as input  ParamDataTypeStr=Inherit: Same as input
  W_wt (pu) : Outport
  T_shaft (pu) : Outport  Port=2
  wires:
  T_wt (pu)/1 -> Sum/1
  Sum2/1 -> Sum/2, Gain/1
  Mutual damping/1 -> Sum2/2
  Sum1/1 -> Mutual damping/1, wbase/1
  Gen speed (pu)/1 -> Sum1/2
  Discrete-Time Integrator/1 -> Sum1/1, W_wt (pu)/1
  1_2H_WT Wind Turbine Inertia Const/1 -> Discrete-Time Integrator/1
  Sum/1 -> 1_2H_WT Wind Turbine Inertia Const/1
  Stiffness Shaft Spring Const/1 -> Sum2/1
  Discrete-Time Integrator1/1 -> Stiffness Shaft Spring Const/1
  wbase/1 -> Discrete-Time Integrator1/1
  Gain/1 -> T_shaft (pu)/1

== system hybrid_fuzzy/Wind/Pitch_angle-controller ==
  wr1 : Inport
  0-pitch_max : Saturate  UpperLimit=45  LowerLimit=0
  Constant2 : Constant  Value=2
  "Rate Limiter   " : RateLimiter  RisingSlewLimit=2  FallingSlewLimit=-2
  Sum : Sum  Inputs=|+-  SaturateOnIntegerOverflow=on
  pitch_gain : Gain  Gain=500  SaturateOnIntegerOverflow=on  OutDataTypeStr=Inherit: Same as input  ParamDataTypeStr=Inherit: Same as input
  Pitch_angle1 : Outport
  wires:
  "Rate Limiter   "/1 -> Pitch_angle1/1
  pitch_gain/1 -> 0-pitch_max/1
  Sum/1 -> pitch_gain/1
  Constant2/1 -> Sum/2
  0-pitch_max/1 -> "Rate Limiter   "/1
  wr1/1 -> Sum/1

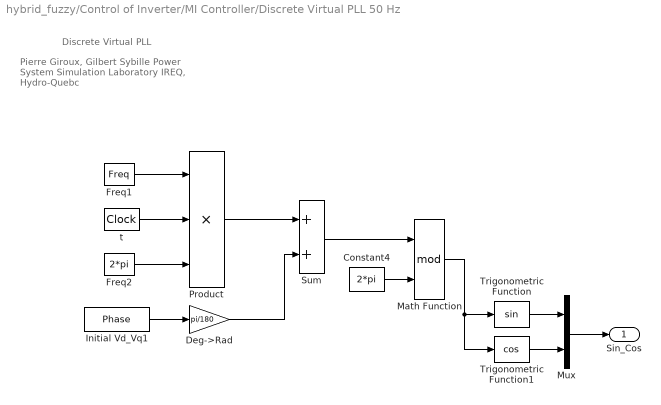
== system hybrid_fuzzy/Control of Inverter/MI Controller/Discrete Virtual PLL 50 Hz ==
  note: Pierre Giroux, Gilbert Sybille
      | Power System Simulation Laboratory
      | IREQ, Hydro-Quebc
  note: Discrete Virtual PLL
  Constant4 : Constant  Value=2*pi
  Deg->Rad : Gain  Gain=pi/180  SaturateOnIntegerOverflow=on  OutDataTypeStr=Inherit: Same as input  ParamDataTypeStr=Inherit: Same as input
  Freq1 : Constant  Value=Freq
  Freq2 : Constant  Value=2*pi
  Initial Vd_Vq1 : Constant  Value=Phase
  Math Function : Math  Operator=mod  SignedPower=on  SaturateOnIntegerOverflow=on
  Mux : Mux  Inputs=2
  Product : Product  Inputs=***  InputSameDT=on  SaturateOnIntegerOverflow=on  OutDataTypeStr=Inherit: Same as first input
  Sum : Sum  InputSameDT=on  SaturateOnIntegerOverflow=on  OutDataTypeStr=Inherit: Same as first input
  Trigonometric Function : Trigonometry
  Trigonometric Function1 : Trigonometry  Operator=cos
  t : DigitalClock  SampleTime=Ts
  Sin_Cos : Outport  VectorParamsAs1DForOutWhenUnconnected=off
  wires:
  Sum/1 -> Math Function/1
  t/1 -> Product/2
  Freq2/1 -> Product/3
  Freq1/1 -> Product/1
  Deg->Rad/1 -> Sum/2
  Initial Vd_Vq1/1 -> Deg->Rad/1
  Product/1 -> Sum/1
  Constant4/1 -> Math Function/2
  Math Function/1 -> Trigonometric Function1/1, Trigonometric Function/1
  Trigonometric Function/1 -> Mux/1
  Trigonometric Function1/1 -> Mux/2
  Mux/1 -> Sin_Cos/1

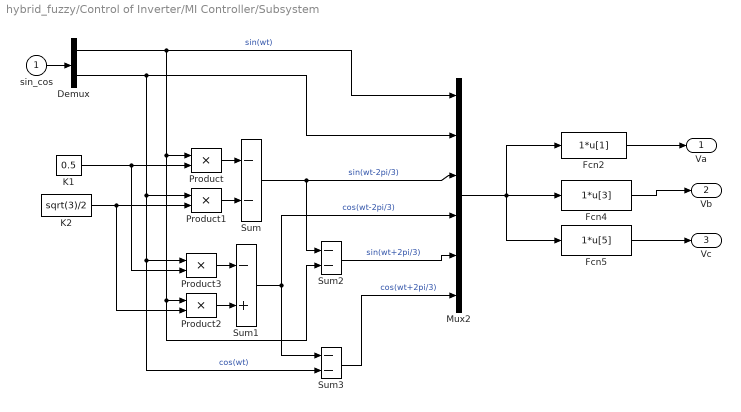
== system hybrid_fuzzy/Control of Inverter/MI Controller/Subsystem ==
  sin_cos : Inport  PortDimensions=2
  Demux : Demux  Outputs=2
      settings: DisplayOption=none
  Fcn2 : Fcn  Expr=1*u[1]
  Fcn4 : Fcn  Expr=1*u[3]
  Fcn5 : Fcn  Expr=1*u[5]
  K1 : Constant  Value=0.5
  K2 : Constant  Value=sqrt(3)/2
  Mux2 : Mux  Inputs=6
  Product{,1..3} (4 alike) : Product  InputSameDT=on  SaturateOnIntegerOverflow=on  OutDataTypeStr=Inherit: Same as first input
  Sum : Sum  Inputs=--  InputSameDT=on  SaturateOnIntegerOverflow=on  OutDataTypeStr=Inherit: Same as first input
  Sum1 : Sum  Inputs=-+  InputSameDT=on  SaturateOnIntegerOverflow=on  OutDataTypeStr=Inherit: Same as first input
  Sum2 : Sum  Inputs=--  InputSameDT=on  SaturateOnIntegerOverflow=on  OutDataTypeStr=Inherit: Same as first input
  Sum3 : Sum  Inputs=--  InputSameDT=on  SaturateOnIntegerOverflow=on  OutDataTypeStr=Inherit: Same as first input
  Va : Outport  VectorParamsAs1DForOutWhenUnconnected=off
  Vb : Outport  Port=2  VectorParamsAs1DForOutWhenUnconnected=off
  Vc : Outport  Port=3  VectorParamsAs1DForOutWhenUnconnected=off
  wires:
  sin_cos/1 -> Demux/1
  Demux/1 -> Product/1, Product2/1, Sum2/2, Mux2/1  "sin(wt)"
  Product/1 -> Sum/1
  Product1/1 -> Sum/2
  Product3/1 -> Sum1/1
  Product2/1 -> Sum1/2
  Sum3/1 -> Mux2/6  "cos(wt+2pi/3)"
  Sum2/1 -> Mux2/5  "sin(wt+2pi/3)"
  K1/1 -> Product/2, Product3/2
  K2/1 -> Product1/2, Product2/2
  Sum/1 -> Mux2/3, Sum2/1  "sin(wt-2pi/3)"
  Sum1/1 -> Mux2/4, Sum3/1  "cos(wt-2pi/3)"
  Demux/2 -> Sum3/2, Product3/1, Product1/1, Mux2/2  "cos(wt)"
  Mux2/1 -> Fcn2/1, Fcn4/1, Fcn5/1
  Fcn2/1 -> Va/1
  Fcn4/1 -> Vb/1
  Fcn5/1 -> Vc/1
